simulink model "AGTF30SysDyn_controlled"  (R2019b)
settings: Solver=ode4  StartTime=0.0  StopTime=MWS.In.t(end)  FixedStep=MWS.In.Ts  RelTol=1e-3  EnableMultiTasking=on
model workspace: external: MAT-File (data not in the file)
values from neighbouring files (symbols this model uses):
  Alpha = [1 2]    [ShiftMap.m]
  MWS =     [MWS.mat]
undefined symbols (not defined in the file or in its folder): K, N, N1sen, N2sen, N3sen, P, T, VAFNdmd, VBVdmd, Wfdmd
libraries: Lib_Cntrl_FirstOrderSensor_TMATS x12, Lib_Solve_ModelSource_TMATS x8, Lib_Cntrl_FirstOrderActuator_TMATS x2, Lib_Solve_OuterLoopIntegrator_TMATS x2, simulink x2, Lib_Solve_IterNRSolverJC_TMATS x1
settings Model: Creator=jwchapm2  LastModifiedBy=jdiegelm
settings DataIOCC: LimitDataPoints=on  SaveFormat=Array  ReturnWorkspaceOutputs=off
settings OptimizationCC: LifeSpan=inf
settings DebuggingCC: SFUnexpectedBacktrackingDiag=warning  SFNoUnconditionalDefaultTransitionDiag=warning  SFExecutionAtInitializationDiag=none  ArithmeticOperatorsInVariantConditions=warning
settings HardwareCC: ProdBitPerPointer=32  ProdBitPerSizeT=32  ProdBitPerPtrDiffT=32  ProdLargestAtomicFloat=None  ProdIntDivRoundTo=Undefined  ProdEndianess=Unspecified  ProdWordSize=32  ProdHWDeviceType=32-bit Generic
settings ModelReferenceCC: PropagateSignalLabelsOutOfModel=off
settings SFSimCC: SimUseLocalCustomCode=off  CustomCodeUndefinedFunction=UseInterfaceOnly
settings RTWCC: RTWUseLocalCustomCode=off
settings CodeAppCC: StateflowObjectComments=on
settings GRTTargetCC: TargetLangStandard=C89/C90 (ANSI)  GeneratePreprocessorConditionals=Disable all
settings ConfigComp: CovMetricSettings=dw  CovHtmlReporting=on  CovSaveCumulativeToWorkspaceVar=on  CovSaveSingleToWorkspaceVar=on  CovExternalEMLEnable=off

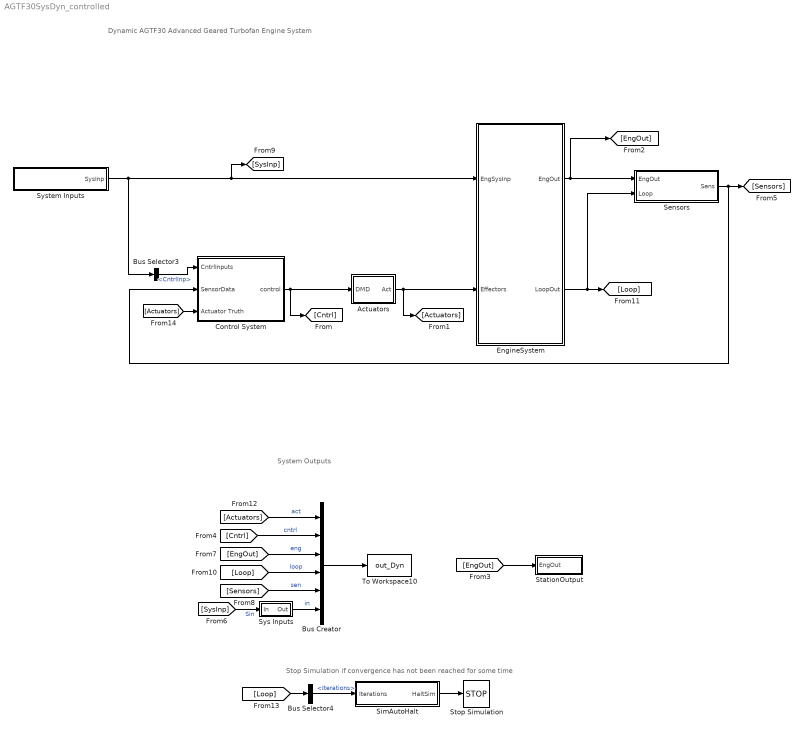
== system AGTF30SysDyn_controlled ==
  note: Stop Simulation if convergence has not been reached for some time
  note: Dynamic AGTF30
      | Advanced Geared Turbofan Engine System
  note: System Outputs
  Actuators : Subsystem
  Bus Creator : BusCreator  Inputs=6
  Bus Selector3 : BusSelector  OutputSignals=CntrlInp
  Bus Selector4 : BusSelector  OutputSignals=Solver.Iterations
  Control System : Subsystem
  EngineSystem : Subsystem
  Sensors : Subsystem
  SimAutoHalt : Subsystem
  StationOutput : Subsystem
  Stop Simulation : Stop
  Sys Inputs : Subsystem
  System Inputs : Subsystem
  To Workspace10 : ToWorkspace  VariableName=out_Dyn  SaveFormat=Timeseries  SampleTime=-1
  wires:
  Actuators/1(Act) -> [Actuators], EngineSystem/2(Effectors)
  Control System/1(control) -> Actuators/1(DMD), [Cntrl]
  Bus Selector3/1 -> Control System/1(CntrlInputs)  "<CntrlInp>"
  System Inputs/1(SysInp) -> Bus Selector3/1, EngineSystem/1(EngSysInp), [SysInp]
  EngineSystem/1(EngOut) -> [EngOut], Sensors/1(EngOut)
  EngineSystem/2(LoopOut) -> Sensors/2(Loop), [Loop]
  [EngOut] -> StationOutput/1(EngOut)
  Bus Creator/1 -> To Workspace10/1
  [Loop] -> Bus Creator/4  "loop"
  [Sensors] -> Bus Creator/5  "sen"
  [EngOut] -> Bus Creator/3  "eng"
  Sys Inputs/1(Out) -> Bus Creator/6  "in"
  [Actuators] -> Bus Creator/1  "act"
  [Cntrl] -> Bus Creator/2  "cntrl"
  Sensors/1(Sens) -> Control System/2(SensorData), [Sensors]
  [Loop] -> Bus Selector4/1
  Bus Selector4/1 -> SimAutoHalt/1(Iterations)  "<Iterations>"
  SimAutoHalt/1(HaltSim) -> Stop Simulation/1
  [SysInp] -> Sys Inputs/1(In)  "Sin"
  [Actuators] -> Control System/3(Actuator Truth)

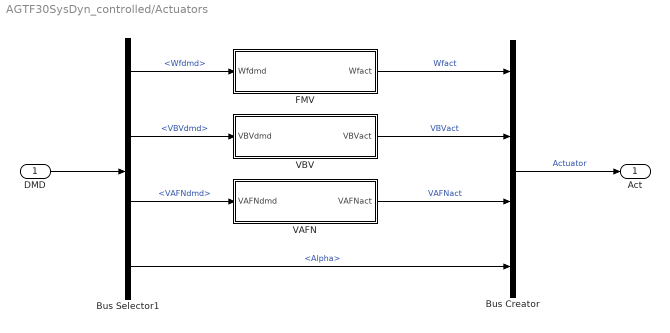
== system AGTF30SysDyn_controlled/Actuators ==
  DMD : Inport
  Bus Creator : BusCreator  Inputs=4
  Bus Selector1 : BusSelector  OutputSignals=Wfdmd,VBVdmd,VAFNdmd,Alpha
  FMV : Subsystem
  VAFN : Subsystem
  VBV : Subsystem
  Act : Outport
  wires:
  DMD/1 -> Bus Selector1/1
  Bus Creator/1 -> Act/1  "Actuator"
  Bus Selector1/3 -> VAFN/1(VAFNdmd)  "<VAFNdmd>"
  Bus Selector1/2 -> VBV/1(VBVdmd)  "<VBVdmd>"
  VBV/1(VBVact) -> Bus Creator/2  "VBVact"
  VAFN/1(VAFNact) -> Bus Creator/3  "VAFNact"
  Bus Selector1/1 -> FMV/1(Wfdmd)  "<Wfdmd>"
  FMV/1(Wfact) -> Bus Creator/1  "Wfact"
  Bus Selector1/4 -> Bus Creator/4  "<Alpha>"

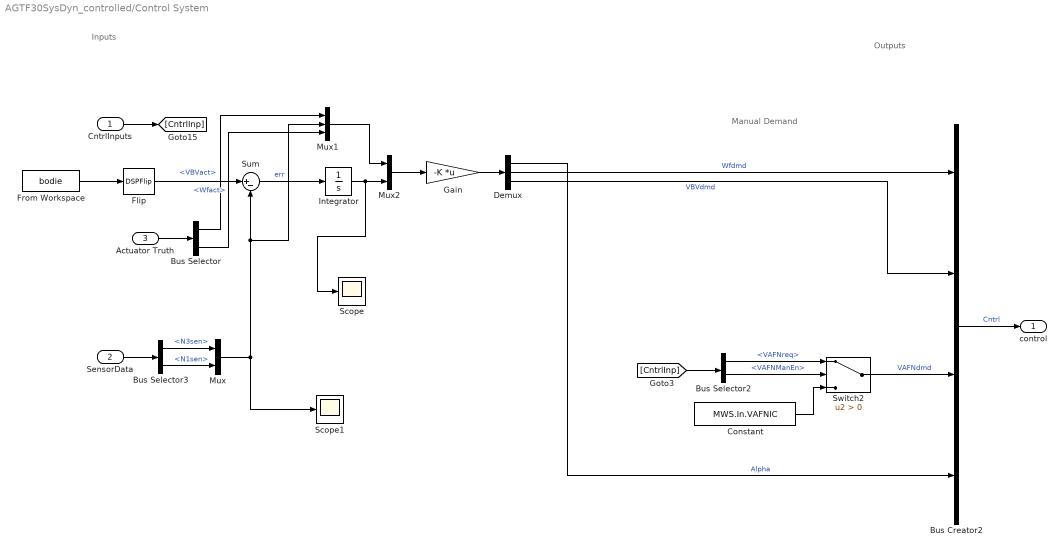
== system AGTF30SysDyn_controlled/Control System ==
  note: Inputs
  note: Outputs
  note: Manual Demand
  CntrlInputs : Inport
  SensorData : Inport  Port=2
  Actuator Truth : Inport  Port=3
  Bus Creator2 : BusCreator  Inputs=Wfdmd,VBVdmd,VAFNdmd,Alpha
  Bus Selector : BusSelector  OutputSignals=VBVact,Wfact
  Bus Selector2 : BusSelector  OutputSignals=ManualOp.VAFNreq,ManualOp.VAFNManEn
  Bus Selector3 : BusSelector  OutputSignals=N.N3sen,N.N1sen
  Constant : Constant  Value=MWS.In.VAFNIC
  Demux : Demux  Outputs=3
  Flip : DSPFlip
  From Workspace : FromWorkspace  VariableName=bodie  SampleTime=0
  Gain : Gain  Gain=-K  Multiplication=Matrix(K*u) (u vector)
  Integrator : Integrator  InitialCondition=[16000 4000]
  Mux : Mux  Inputs=2
  Mux1 : Mux  Inputs=3
  Mux2 : Mux  Inputs=2
  Scope : Scope
  Scope1 : Scope
  Sum : Sum  Inputs=|+-
  Switch2 : Switch  Criteria=u2 > Threshold
  control : Outport
  wires:
  CntrlInputs/1 -> [CntrlInp]
  Switch2/1 -> Bus Creator2/3  "VAFNdmd"
  SensorData/1 -> Bus Selector3/1
  Bus Creator2/1 -> control/1  "Cntrl"
  Bus Selector2/1 -> Switch2/1  "<VAFNreq>"
  [CntrlInp] -> Bus Selector2/1
  Bus Selector2/2 -> Switch2/2  "<VAFNManEn>"
  Constant/1 -> Switch2/3
  Bus Selector3/2 -> Mux/2  "<N1sen>"
  Bus Selector3/1 -> Mux/1  "<N3sen>"
  Mux/1 -> Scope1/1, Mux1/2, Sum/2
  Sum/1 -> Integrator/1  "err"
  Demux/2 -> Bus Creator2/1  "Wfdmd"
  Demux/1 -> Bus Creator2/4  "Alpha"
  Demux/3 -> Bus Creator2/2  "VBVdmd"
  Gain/1 -> Demux/1
  Actuator Truth/1 -> Bus Selector/1
  Bus Selector/2 -> Mux1/3  "<Wfact>"
  Bus Selector/1 -> Mux1/1  "<VBVact>"
  Flip/1 -> Sum/1
  Mux2/1 -> Gain/1
  Integrator/1 -> Scope/1, Mux2/2
  Mux1/1 -> Mux2/1
  From Workspace/1 -> Flip/1

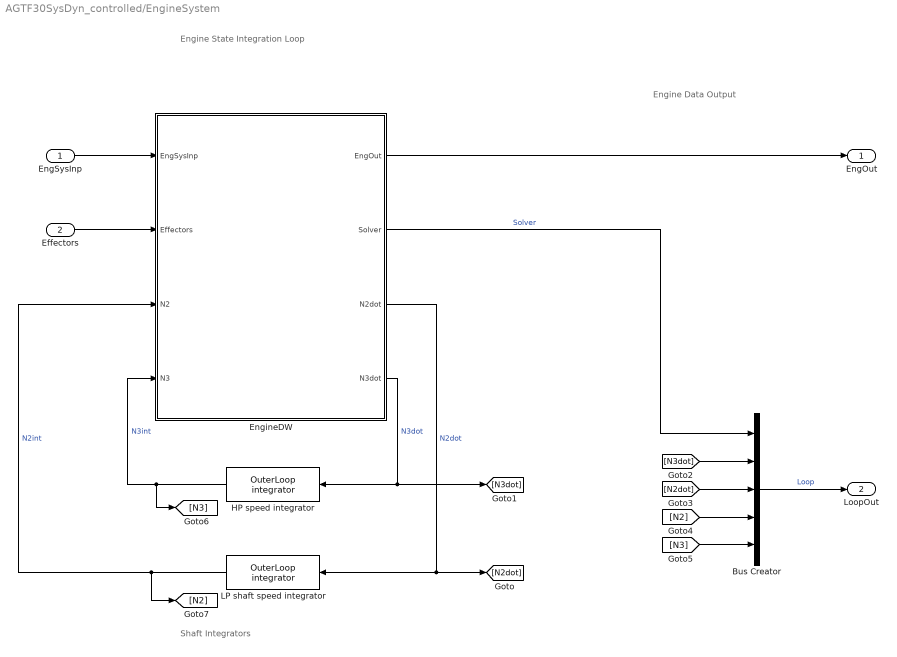
== system AGTF30SysDyn_controlled/EngineSystem ==
  note: Shaft Integrators
  note: Engine State
      | Integration Loop
  note: Engine Data Output
  EngSysInp : Inport
  Effectors : Inport  Port=2
  Bus Creator : BusCreator  Inputs=5
  EngineDW : Subsystem
  HP speed integrator : Lib_Solve_OuterLoopIntegrator_TMATS/OuterLoop integrator  OL_IC_M=MWS.In.N3IC
  LP shaft speed integrator : Lib_Solve_OuterLoopIntegrator_TMATS/OuterLoop integrator  OL_IC_M=MWS.In.N2IC
  EngOut : Outport
  LoopOut : Outport  Port=2
  wires:
  EngSysInp/1 -> EngineDW/1(EngSysInp)
  LP shaft speed integrator/1 -> [N2], EngineDW/3(N2)  "N2int"
  Effectors/1 -> EngineDW/2(Effectors)
  EngineDW/3(N2dot) -> LP shaft speed integrator/1, [N2dot]  "N2dot"
  EngineDW/2(Solver) -> Bus Creator/1  "Solver"
  EngineDW/1(EngOut) -> EngOut/1
  EngineDW/4(N3dot) -> HP speed integrator/1, [N3dot]  "N3dot"
  HP speed integrator/1 -> [N3], EngineDW/4(N3)  "N3int"
  Bus Creator/1 -> LoopOut/1  "Loop"
  [N3dot] -> Bus Creator/2
  [N2dot] -> Bus Creator/3
  [N2] -> Bus Creator/4
  [N3] -> Bus Creator/5

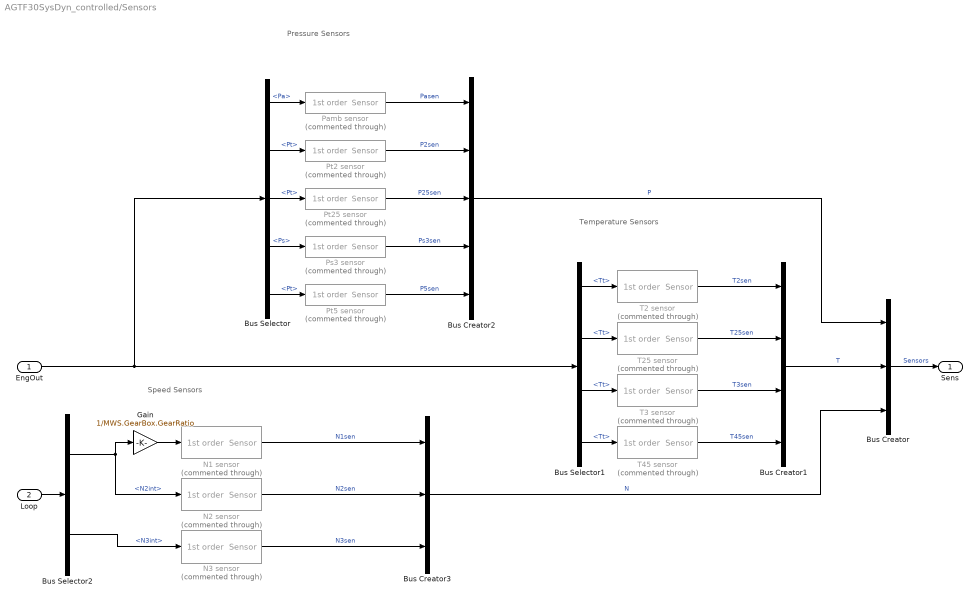
== system AGTF30SysDyn_controlled/Sensors ==
  note: Pressure Sensors
  note: Temperature Sensors
  note: Speed Sensors
  EngOut : Inport
  Loop : Inport  Port=2
  Bus Creator : BusCreator  Inputs=P,T,N
  Bus Creator1 : BusCreator  Inputs=4
  Bus Creator2 : BusCreator  Inputs=5
  Bus Creator3 : BusCreator  Inputs=N1sen,N2sen,N3sen
  Bus Selector : BusSelector  OutputSignals=Amb.Pa,S2.Pt,S25.Pt,S36.Ps,S5.Pt
  Bus Selector1 : BusSelector  OutputSignals=S2.Tt,S25.Tt,S36.Tt,S45.Tt
  Bus Selector2 : BusSelector  OutputSignals=N2int,N3int
  Gain : Gain  Gain=1/MWS.GearBox.GearRatio
  N1 sensor : Lib_Cntrl_FirstOrderSensor_TMATS/1st order  Sensor  Commented=through  IC_M=MWS.In.Sensor.ICN1  Sen_Max_M=MWS.Sensor.N1.Max  Sen_Min_M=MWS.Sensor.N1.Min  Gain_M=1  Tau_M=MWS.Sensor.N1.Tau  GN_EN_M=off  GN_NST_M=MWS.In.Ts  GN_C_M=1  GN_MinNoise_M=0.3  F_Gain_M=1  F_Drift_M=0
  N2 sensor : Lib_Cntrl_FirstOrderSensor_TMATS/1st order  Sensor  Commented=through  IC_M=MWS.In.Sensor.ICN2  Sen_Max_M=MWS.Sensor.N2.Max  Sen_Min_M=MWS.Sensor.N2.Min  Gain_M=1  Tau_M=MWS.Sensor.N2.Tau  GN_EN_M=off  GN_NST_M=MWS.In.Ts  GN_C_M=1  GN_MinNoise_M=0.3  F_Gain_M=1  F_Drift_M=0
  N3 sensor : Lib_Cntrl_FirstOrderSensor_TMATS/1st order  Sensor  Commented=through  IC_M=MWS.In.Sensor.ICN3  Sen_Max_M=MWS.Sensor.N3.Max  Sen_Min_M=MWS.Sensor.N3.Min  Gain_M=1  Tau_M=MWS.Sensor.N3.Tau  GN_EN_M=off  GN_NST_M=MWS.In.Ts  GN_C_M=1  GN_MinNoise_M=0.3  F_Gain_M=1  F_Drift_M=0
  Pamb sensor : Lib_Cntrl_FirstOrderSensor_TMATS/1st order  Sensor  Commented=through  IC_M=MWS.In.Sensor.ICPa  Sen_Max_M=MWS.Sensor.P2.Max  Sen_Min_M=MWS.Sensor.P2.Min  Gain_M=1  Tau_M=MWS.Sensor.P2.Tau  GN_EN_M=off  GN_NST_M=MWS.In.Ts  GN_C_M=1  GN_MinNoise_M=0.3  F_Gain_M=1  F_Drift_M=0
  Ps3 sensor : Lib_Cntrl_FirstOrderSensor_TMATS/1st order  Sensor  Commented=through  IC_M=MWS.In.Sensor.ICPs3  Sen_Max_M=MWS.Sensor.Ps3.Max  Sen_Min_M=MWS.Sensor.Ps3.Min  Gain_M=1  Tau_M=MWS.Sensor.Ps3.Tau  GN_EN_M=off  GN_NST_M=MWS.In.Ts  GN_C_M=1  GN_MinNoise_M=0.3  F_Gain_M=1  F_Drift_M=0
  Pt2 sensor : Lib_Cntrl_FirstOrderSensor_TMATS/1st order  Sensor  Commented=through  IC_M=MWS.In.Sensor.ICP2  Sen_Max_M=MWS.Sensor.P2.Max  Sen_Min_M=MWS.Sensor.P2.Min  Gain_M=1  Tau_M=MWS.Sensor.P2.Tau  GN_EN_M=off  GN_NST_M=MWS.In.Ts  GN_C_M=1  GN_MinNoise_M=0.3  F_Gain_M=1  F_Drift_M=0
  Pt25 sensor : Lib_Cntrl_FirstOrderSensor_TMATS/1st order  Sensor  Commented=through  IC_M=MWS.In.Sensor.ICP25  Sen_Max_M=MWS.Sensor.P25.Max  Sen_Min_M=MWS.Sensor.P25.Min  Gain_M=1  Tau_M=MWS.Sensor.P25.Tau  GN_EN_M=off  GN_NST_M=MWS.In.Ts  GN_C_M=1  GN_MinNoise_M=0.3  F_Gain_M=1  F_Drift_M=0
  Pt5 sensor : Lib_Cntrl_FirstOrderSensor_TMATS/1st order  Sensor  Commented=through  IC_M=MWS.In.Sensor.ICP5  Sen_Max_M=MWS.Sensor.P5.Max  Sen_Min_M=MWS.Sensor.P5.Min  Gain_M=1  Tau_M=MWS.Sensor.P5.Tau  GN_EN_M=off  GN_NST_M=MWS.In.Ts  GN_C_M=1  GN_MinNoise_M=0.3  F_Gain_M=1  F_Drift_M=0
  T2 sensor : Lib_Cntrl_FirstOrderSensor_TMATS/1st order  Sensor  Commented=through  IC_M=MWS.In.Sensor.ICT2  Sen_Max_M=MWS.Sensor.T2.Max  Sen_Min_M=MWS.Sensor.T2.Min  Gain_M=1  Tau_M=MWS.Sensor.T2.Tau  GN_EN_M=off  GN_NST_M=MWS.In.Ts  GN_C_M=1  GN_MinNoise_M=0.3  F_Gain_M=1  F_Drift_M=0
  T25 sensor : Lib_Cntrl_FirstOrderSensor_TMATS/1st order  Sensor  Commented=through  IC_M=MWS.In.Sensor.ICT25  Sen_Max_M=MWS.Sensor.T25.Max  Sen_Min_M=MWS.Sensor.T25.Min  Gain_M=1  Tau_M=MWS.Sensor.T25.Tau  GN_EN_M=off  GN_NST_M=MWS.In.Ts  GN_C_M=1  GN_MinNoise_M=0.3  F_Gain_M=1  F_Drift_M=0
  T3 sensor : Lib_Cntrl_FirstOrderSensor_TMATS/1st order  Sensor  Commented=through  IC_M=MWS.In.Sensor.ICT3  Sen_Max_M=MWS.Sensor.T3.Max  Sen_Min_M=MWS.Sensor.T3.Min  Gain_M=1  Tau_M=MWS.Sensor.T3.Tau  GN_EN_M=off  GN_NST_M=MWS.In.Ts  GN_C_M=1  GN_MinNoise_M=0.3  F_Gain_M=1  F_Drift_M=0
  T45 sensor : Lib_Cntrl_FirstOrderSensor_TMATS/1st order  Sensor  Commented=through  IC_M=MWS.In.Sensor.ICT45  Sen_Max_M=MWS.Sensor.T45.Max*10  Sen_Min_M=MWS.Sensor.T45.Min  Gain_M=1  Tau_M=MWS.Sensor.T45.Tau  GN_EN_M=off  GN_NST_M=MWS.In.Ts  GN_C_M=1  GN_MinNoise_M=0.3  F_Gain_M=1  F_Drift_M=0
  Sens : Outport
  wires:
  Bus Creator/1 -> Sens/1  "Sensors"
  Bus Selector/2 -> Pt2 sensor/1  "<Pt>"
  Bus Creator2/1 -> Bus Creator/1  "P"
  Bus Creator1/1 -> Bus Creator/2  "T"
  Bus Selector1/1 -> T2 sensor/1  "<Tt>"
  Bus Creator3/1 -> Bus Creator/3  "N"
  Bus Selector/3 -> Pt25 sensor/1  "<Pt>"
  Bus Selector/5 -> Pt5 sensor/1  "<Pt>"
  Pt2 sensor/1 -> Bus Creator2/2  "P2sen"
  Pt25 sensor/1 -> Bus Creator2/3  "P25sen"
  Pt5 sensor/1 -> Bus Creator2/5  "P5sen"
  Bus Selector1/2 -> T25 sensor/1  "<Tt>"
  Bus Selector1/3 -> T3 sensor/1  "<Tt>"
  Bus Selector1/4 -> T45 sensor/1  "<Tt>"
  T2 sensor/1 -> Bus Creator1/1  "T2sen"
  T25 sensor/1 -> Bus Creator1/2  "T25sen"
  T3 sensor/1 -> Bus Creator1/3  "T3sen"
  N1 sensor/1 -> Bus Creator3/1  "N1sen"
  Bus Selector/4 -> Ps3 sensor/1  "<Ps>"
  N3 sensor/1 -> Bus Creator3/3  "N3sen"
  Bus Selector/1 -> Pamb sensor/1  "<Pa>"
  Pamb sensor/1 -> Bus Creator2/1  "Pasen"
  N2 sensor/1 -> Bus Creator3/2  "N2sen"
  EngOut/1 -> Bus Selector/1, Bus Selector1/1
  Bus Selector2/2 -> N3 sensor/1  "<N3int>"
  Bus Selector2/1 -> N2 sensor/1, Gain/1  "<N2int>"
  Gain/1 -> N1 sensor/1
  Loop/1 -> Bus Selector2/1
  T45 sensor/1 -> Bus Creator1/4  "T45sen"
  Ps3 sensor/1 -> Bus Creator2/4  "Ps3sen"

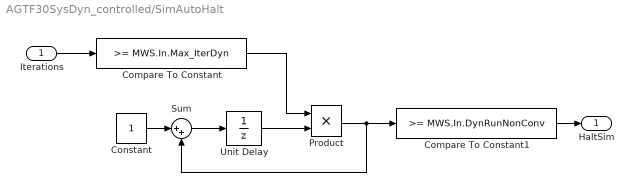
== system AGTF30SysDyn_controlled/SimAutoHalt ==
  Iterations : Inport
  Compare To Constant : simulink/Logic and Bit Operations/Compare To Constant  relop=>=  const=MWS.In.Max_IterDyn  OutDataTypeStr=boolean
  Compare To Constant1 : simulink/Logic and Bit Operations/Compare To Constant  relop=>=  const=MWS.In.DynRunNonConv  OutDataTypeStr=boolean
  Constant : Constant
  Product : Product
  Sum : Sum  Inputs=|++
  Unit Delay : UnitDelay  SampleTime=-1  HasFrameUpgradeWarning=on
  HaltSim : Outport
  wires:
  Compare To Constant1/1 -> HaltSim/1
  Iterations/1 -> Compare To Constant/1
  Compare To Constant/1 -> Product/1
  Constant/1 -> Sum/1
  Sum/1 -> Unit Delay/1
  Unit Delay/1 -> Product/2
  Product/1 -> Sum/2, Compare To Constant1/1

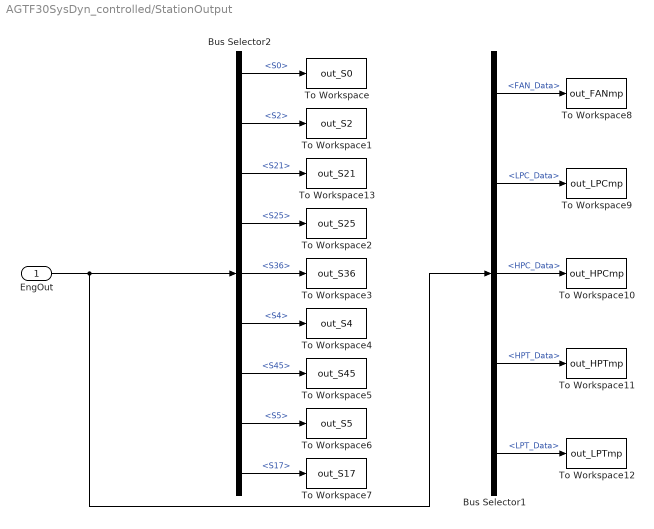
== system AGTF30SysDyn_controlled/StationOutput ==
  EngOut : Inport
  Bus Selector1 : BusSelector  OutputSignals=Data.FAN_Data,Data.LPC_Data,Data.HPC_Data,Data.HPT_Data,Data.LPT_Data
  Bus Selector2 : BusSelector  OutputSignals=S0,S2,S21,S25,S36,S4,S45,S5,S17
  To Workspace : ToWorkspace  VariableName=out_S0  SaveFormat=Timeseries  SampleTime=-1
  To Workspace1 : ToWorkspace  VariableName=out_S2  SaveFormat=Timeseries  SampleTime=-1
  To Workspace10 : ToWorkspace  VariableName=out_HPCmp  SaveFormat=Timeseries  SampleTime=-1
  To Workspace11 : ToWorkspace  VariableName=out_HPTmp  SaveFormat=Timeseries  SampleTime=-1
  To Workspace12 : ToWorkspace  VariableName=out_LPTmp  SaveFormat=Timeseries  SampleTime=-1
  To Workspace13 : ToWorkspace  VariableName=out_S21  SaveFormat=Timeseries  SampleTime=-1
  To Workspace2 : ToWorkspace  VariableName=out_S25  SaveFormat=Timeseries  SampleTime=-1
  To Workspace3 : ToWorkspace  VariableName=out_S36  SaveFormat=Timeseries  SampleTime=-1
  To Workspace4 : ToWorkspace  VariableName=out_S4  SaveFormat=Timeseries  SampleTime=-1
  To Workspace5 : ToWorkspace  VariableName=out_S45  SaveFormat=Timeseries  SampleTime=-1
  To Workspace6 : ToWorkspace  VariableName=out_S5  SaveFormat=Timeseries  SampleTime=-1
  To Workspace7 : ToWorkspace  VariableName=out_S17  SaveFormat=Timeseries  SampleTime=-1
  To Workspace8 : ToWorkspace  VariableName=out_FANmp  SaveFormat=Timeseries  SampleTime=-1
  To Workspace9 : ToWorkspace  VariableName=out_LPCmp  SaveFormat=Timeseries  SampleTime=-1
  wires:
  Bus Selector2/3 -> To Workspace13/1  "<S21>"
  Bus Selector2/1 -> To Workspace/1  "<S0>"
  EngOut/1 -> Bus Selector1/1, Bus Selector2/1
  Bus Selector2/2 -> To Workspace1/1  "<S2>"
  Bus Selector2/4 -> To Workspace2/1  "<S25>"
  Bus Selector2/5 -> To Workspace3/1  "<S36>"
  Bus Selector2/6 -> To Workspace4/1  "<S4>"
  Bus Selector2/7 -> To Workspace5/1  "<S45>"
  Bus Selector2/8 -> To Workspace6/1  "<S5>"
  Bus Selector2/9 -> To Workspace7/1  "<S17>"
  Bus Selector1/1 -> To Workspace8/1  "<FAN_Data>"
  Bus Selector1/2 -> To Workspace9/1  "<LPC_Data>"
  Bus Selector1/3 -> To Workspace10/1  "<HPC_Data>"
  Bus Selector1/4 -> To Workspace11/1  "<HPT_Data>"
  Bus Selector1/5 -> To Workspace12/1  "<LPT_Data>"

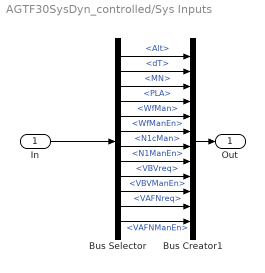
== system AGTF30SysDyn_controlled/Sys Inputs ==
  In : Inport
  Bus Creator1 : BusCreator  Inputs=12
  Bus Selector : BusSelector  OutputSignals=Env.Alt,Env.dT,Env.MN,CntrlInp.PLA,CntrlInp.ManualOp.WfMan,CntrlInp.ManualOp.WfManEn,CntrlInp.ManualOp.N1cMan,CntrlInp.ManualOp.N1ManEn,CntrlInp.ManualOp.VBVreq,CntrlInp.ManualOp.VBVManEn,CntrlInp.ManualOp.VAFNreq,CntrlInp.ManualOp.VAFNManEn
  Out : Outport
  wires:
  In/1 -> Bus Selector/1
  Bus Selector/4 -> Bus Creator1/4  "<PLA>"
  Bus Selector/6 -> Bus Creator1/6  "<WfManEn>"
  Bus Selector/7 -> Bus Creator1/7  "<N1cMan>"
  Bus Selector/8 -> Bus Creator1/8  "<N1ManEn>"
  Bus Selector/9 -> Bus Creator1/9  "<VBVreq>"
  Bus Selector/10 -> Bus Creator1/10  "<VBVManEn>"
  Bus Selector/11 -> Bus Creator1/11  "<VAFNreq>"
  Bus Selector/3 -> Bus Creator1/3  "<MN>"
  Bus Selector/5 -> Bus Creator1/5  "<WfMan>"
  Bus Selector/1 -> Bus Creator1/1  "<Alt>"
  Bus Selector/12 -> Bus Creator1/12  "<VAFNManEn>"
  Bus Selector/2 -> Bus Creator1/2  "<dT>"
  Bus Creator1/1 -> Out/1

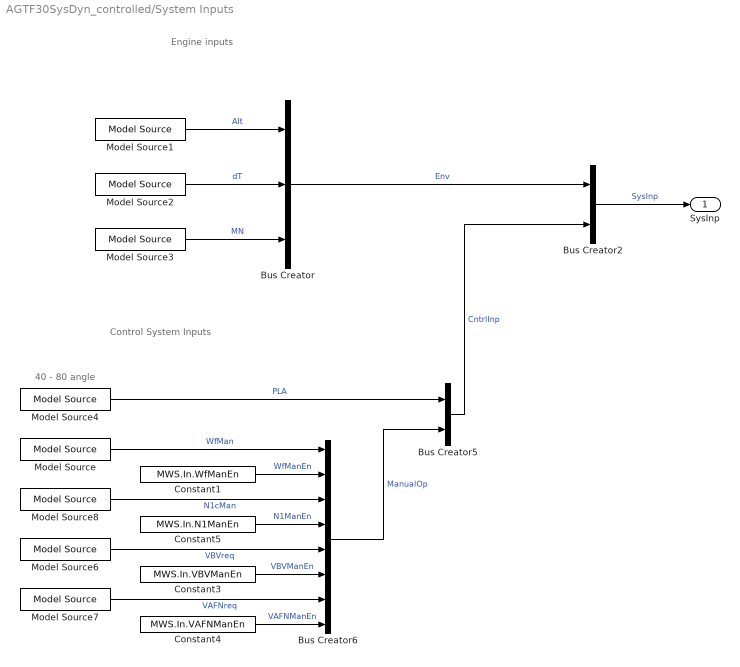
== system AGTF30SysDyn_controlled/System Inputs ==
  note: Engine inputs
  note: Control System Inputs
  note: 40 - 80 angle
  Bus Creator : BusCreator  Inputs=3
  Bus Creator2 : BusCreator  Inputs=2
  Bus Creator5 : BusCreator  Inputs=2
  Bus Creator6 : BusCreator  Inputs=8
  Constant1 : Constant  Value=MWS.In.WfManEn
  Constant3 : Constant  Value=MWS.In.VBVManEn
  Constant4 : Constant  Value=MWS.In.VAFNManEn
  Constant5 : Constant  Value=MWS.In.N1ManEn
  Model Source : Lib_Solve_ModelSource_TMATS/Model Source  T_vec_M=MWS.In.Wfreq(2,:)  input_array_M=MWS.In.Wfreq(1,:)
  Model Source1 : Lib_Solve_ModelSource_TMATS/Model Source  T_vec_M=MWS.In.Alt(2,:)  input_array_M=MWS.In.Alt(1,:)
  Model Source2 : Lib_Solve_ModelSource_TMATS/Model Source  T_vec_M=MWS.In.dT(2,:)  input_array_M=MWS.In.dT(1,:)
  Model Source3 : Lib_Solve_ModelSource_TMATS/Model Source  T_vec_M=MWS.In.MN(2,:)  input_array_M=MWS.In.MN(1,:)
  Model Source4 : Lib_Solve_ModelSource_TMATS/Model Source  T_vec_M=MWS.In.PLA(2,:)  input_array_M=MWS.In.PLA(1,:)
  Model Source6 : Lib_Solve_ModelSource_TMATS/Model Source  T_vec_M=MWS.In.VBVreq(2,:)  input_array_M=MWS.In.VBVreq(1,:)
  Model Source7 : Lib_Solve_ModelSource_TMATS/Model Source  T_vec_M=MWS.In.VAFNreq(2,:)  input_array_M=MWS.In.VAFNreq(1,:)
  Model Source8 : Lib_Solve_ModelSource_TMATS/Model Source  T_vec_M=MWS.In.N1creq(2,:)  input_array_M=MWS.In.N1creq(1,:)
  SysInp : Outport
  wires:
  Model Source1/1 -> Bus Creator/1  "Alt"
  Model Source2/1 -> Bus Creator/2  "dT"
  Model Source3/1 -> Bus Creator/3  "MN"
  Bus Creator/1 -> Bus Creator2/1  "Env"
  Bus Creator5/1 -> Bus Creator2/2  "CntrlInp"
  Bus Creator2/1 -> SysInp/1  "SysInp"
  Model Source6/1 -> Bus Creator6/5  "VBVreq"
  Model Source7/1 -> Bus Creator6/7  "VAFNreq"
  Model Source4/1 -> Bus Creator5/1  "PLA"
  Bus Creator6/1 -> Bus Creator5/2  "ManualOp"
  Model Source/1 -> Bus Creator6/1  "WfMan"
  Constant1/1 -> Bus Creator6/2  "WfManEn"
  Constant4/1 -> Bus Creator6/8  "VAFNManEn"
  Constant3/1 -> Bus Creator6/6  "VBVManEn"
  Model Source8/1 -> Bus Creator6/3  "N1cMan"
  Constant5/1 -> Bus Creator6/4  "N1ManEn"

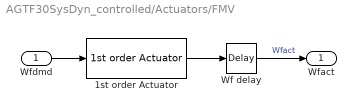
== system AGTF30SysDyn_controlled/Actuators/FMV ==
  Wfdmd : Inport
  1st order Actuator : Lib_Cntrl_FirstOrderActuator_TMATS/1st order Actuator  Gain_M=MWS.Act.FMV.Gain  Tau_M=MWS.Act.FMV.Tau  IC_M=MWS.In.WfIC  MaxSat_M=MWS.Act.FMV.max  MinSat_M=MWS.Act.FMV.min  deadband_M=0.0  rateLimit_M=MWS.Act.FMV.rateLimit
  Wf delay : TransportDelay  DelayTime=MWS.Act.FMV.TWf_dly  InitialOutput=MWS.In.WfIC
  Wfact : Outport
  wires:
  Wf delay/1 -> Wfact/1  "Wfact"
  Wfdmd/1 -> 1st order Actuator/1
  1st order Actuator/1 -> Wf delay/1

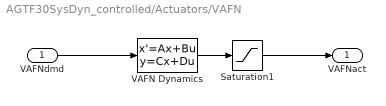
== system AGTF30SysDyn_controlled/Actuators/VAFN ==
  VAFNdmd : Inport
  Saturation1 : Saturate  UpperLimit=MWS.Act.VAFN_max  LowerLimit=0  LinearizeAsGain=off
  VAFN Dynamics : StateSpace  A=MWS.Act.VAFN.A  B=MWS.Act.VAFN.B  C=MWS.Act.VAFN.C  D=MWS.Act.VAFN.D  InitialCondition=MWS.In.VAFNIC
  VAFNact : Outport
  wires:
  Saturation1/1 -> VAFNact/1
  VAFNdmd/1 -> VAFN Dynamics/1
  VAFN Dynamics/1 -> Saturation1/1

== system AGTF30SysDyn_controlled/Actuators/VBV ==
  VBVdmd : Inport
  1st order Actuator : Lib_Cntrl_FirstOrderActuator_TMATS/1st order Actuator  Gain_M=MWS.Act.VBV.Gain  Tau_M=MWS.Act.VBV.Tau  IC_M=MWS.In.VBVIC  MaxSat_M=MWS.Act.VBV.max  MinSat_M=MWS.Act.VBV.min  deadband_M=0.0  rateLimit_M=100000
  VBVact : Outport
  wires:
  VBVdmd/1 -> 1st order Actuator/1
  1st order Actuator/1 -> VBVact/1  "VBVact"

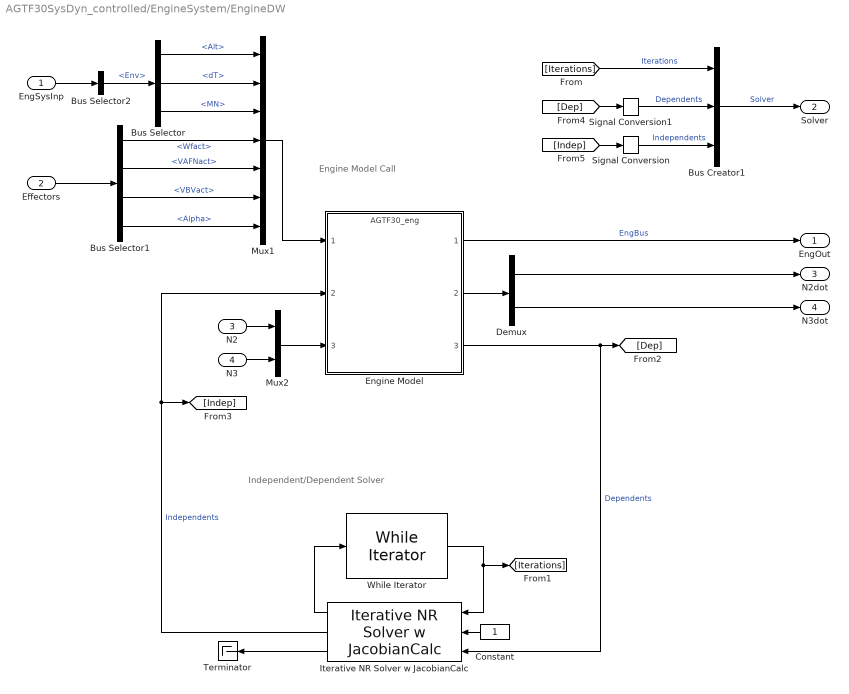
== system AGTF30SysDyn_controlled/EngineSystem/EngineDW ==
  note: Independent/Dependent Solver
  note: Engine Model Call
  EngSysInp : Inport
  Effectors : Inport  Port=2
  N2 : Inport  Port=3
  N3 : Inport  Port=4
  Bus Creator1 : BusCreator  Inputs=3
  Bus Selector : BusSelector  OutputSignals=Alt,dT,MN
  Bus Selector1 : BusSelector  OutputSignals=Wfact,VAFNact,VBVact,Alpha
  Bus Selector2 : BusSelector  OutputSignals=Env
  Constant : Constant
  Demux : Demux  Outputs=2
  Engine Model : ModelReference  ModelNameDialog=AGTF30_eng.mdl  SimulationMode=Normal  ModelReferenceVersion=1.306
  Iterative NR Solver w JacobianCalc : Lib_Solve_IterNRSolverJC_TMATS/Iterative NR Solver w JacobianCalc  SJac_Per_M=MWS.In.JPerDyn  SNR_IC_M=MWS.In.ICcom  SNR_DX_M=MWS.In.dX  SNR_Mx_M=100000  SNR_Mn_M=0.0001  SJacobianAttempts_M=MWS.In.NRADyn  Cond_Limits_M=MWS.In.Lim
  Mux1 : Mux  Inputs=7
  Mux2 : Mux  Inputs=2
  Signal Conversion : SignalConversion  OverrideOpt=off
  Signal Conversion1 : SignalConversion  OverrideOpt=off
  Terminator : Terminator
  While Iterator : WhileIterator  MaxIters=MWS.In.Max_IterDyn  WhileBlockType=do-while  ShowIterationPort=on
  EngOut : Outport
  Solver : Outport  Port=2
  N2dot : Outport  Port=3
  N3dot : Outport  Port=4
  wires:
  Engine Model/1 -> EngOut/1  "EngBus"
  Mux1/1 -> Engine Model/1
  EngSysInp/1 -> Bus Selector2/1
  Effectors/1 -> Bus Selector1/1
  Constant/1 -> Iterative NR Solver w JacobianCalc/2
  Iterative NR Solver w JacobianCalc/2 -> Engine Model/2, [Indep]  "Independents"
  Engine Model/3 -> Iterative NR Solver w JacobianCalc/3, [Dep]  "Dependents"
  While Iterator/1 -> [Iterations], Iterative NR Solver w JacobianCalc/1
  Iterative NR Solver w JacobianCalc/1 -> While Iterator/1
  Engine Model/2 -> Demux/1
  Mux2/1 -> Engine Model/3
  Iterative NR Solver w JacobianCalc/3 -> Terminator/1
  N2/1 -> Mux2/1
  N3/1 -> Mux2/2
  Demux/1 -> N2dot/1
  Demux/2 -> N3dot/1
  Bus Selector/1 -> Mux1/1  "<Alt>"
  Bus Selector/2 -> Mux1/2  "<dT>"
  Bus Selector/3 -> Mux1/3  "<MN>"
  Bus Selector1/3 -> Mux1/6  "<VBVact>"
  Bus Selector1/1 -> Mux1/4  "<Wfact>"
  [Iterations] -> Bus Creator1/1  "Iterations"
  Bus Creator1/1 -> Solver/1  "Solver"
  [Dep] -> Signal Conversion1/1
  [Indep] -> Signal Conversion/1
  Signal Conversion/1 -> Bus Creator1/3  "Independents"
  Signal Conversion1/1 -> Bus Creator1/2  "Dependents"
  Bus Selector1/2 -> Mux1/5  "<VAFNact>"
  Bus Selector2/1 -> Bus Selector/1  "<Env>"
  Bus Selector1/4 -> Mux1/7  "<Alpha>"
